simulink model "UDP_Receive_Expanded"  (Simulink 8.3)
settings: Solver=ode45  StartTime=0.0  StopTime=inf  RelTol=1e-3
libraries: simulink x1, dspnetwork x1
settings Model: Creator=Drudoo  LastModifiedBy=Drudoo
settings DataIOCC: SignalLoggingSaveFormat=Dataset
settings DebuggingCC: UnderspecifiedInitializationDetection=Simplified  StateNameClashWarn=none
settings GRTTargetCC: CombineOutputUpdateFcns=on  GRTInterface=off

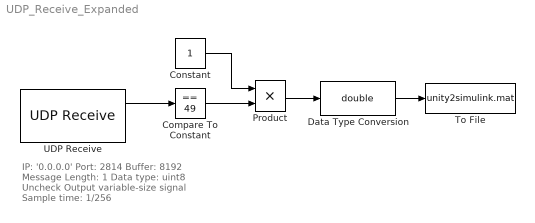
== system UDP_Receive_Expanded ==
  note: IP: '0.0.0.0'
      | Port: 2814
      | Buffer: 8192
      | Message Length: 1
      | Data type: uint8
      | Uncheck Output variable-size signal
      | Sample time: 1/256
  Compare To Constant : simulink/Logic and Bit Operations/Compare To Constant  relop===  const=49  OutDataTypeStr=boolean
  "Constant " : Constant
  "Data Type Conversion " : DataTypeConversion  OutDataTypeStr=double
  Product : Product  RndMeth=Zero
  To File : ToFile  Filename=unity2simulink.mat  SampleTime=1/256
  UDP Receive : dspnetwork/UDP Receive  localURL='0.0.0.0'  localPort=2814  remoteURL='0.0.0.0'  remotePort=-1  recvBufferSize=8192  dims=1  signalDatatype=uint8  isVarSize=off  showBlockingTime=off  blockingTime=0  sampletime=1/256
  wires:
  "Data Type Conversion "/1 -> To File/1
  "Constant "/1 -> Product/1
  Compare To Constant/1 -> Product/2
  Product/1 -> "Data Type Conversion "/1
  UDP Receive/1 -> Compare To Constant/1
